simulink model "Simu_Autopilot_2015_updated"  (R2015a)
settings: Solver=ode15s  StartTime=0.0  StopTime=240  RelTol=1e-3
InitFcn:
  | clear all
  | addpath('../parameters/')
  | aircraft_parameters
  | simulation_parameters
  | wind_parameters
  | compute_autopilot_gains
undefined symbols (not defined in the file or in its folder): autopilot, drawAircraft, forces_moments, path_follow, path_manager, plotmavstatevariables, SIM, UAV, WIND
libraries: simulink x4
settings Model: CovHtmlReporting=off  CovSFcnEnable=off  Creator=beard  LastModifiedBy=User
settings DataIOCC: SignalLoggingSaveFormat=ModelDataLogs
settings OptimizationCC: ExpressionDepthLimit=2147483647  InitFltsAndDblsToZero=on
settings DebuggingCC: UnderspecifiedInitializationDetection=Classic  MergeDetectMultiDrivingBlocksExec=none  SolverPrmCheckMsg=warning  FcnCallInpInsideContextMsg=EnableAllAsWarning  StateNameClashWarn=warning
settings GRTTargetCC: CombineOutputUpdateFcns=off  GRTInterface=on

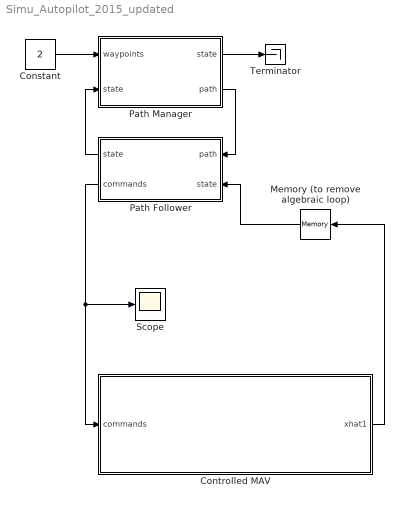
== system Simu_Autopilot_2015_updated ==
  Constant : Constant  Value=2
  Controlled MAV : Subsystem
  Memory (to remove algebraic loop) : Memory
  Path Follower : Subsystem
  Path Manager : Subsystem
  Scope : Scope
  Terminator : Terminator
  wires:
  Controlled MAV/1(xhat1) -> Memory (to remove algebraic loop)/1
  Memory (to remove algebraic loop)/1 -> Path Follower/2(state)
  Path Follower/2(commands) -> Scope/1, Controlled MAV/1(commands)
  Path Follower/1("state ") -> Path Manager/2(state)
  Path Manager/2(path) -> Path Follower/1(path)
  Constant/1 -> Path Manager/1(waypoints)
  Path Manager/1("state ") -> Terminator/1

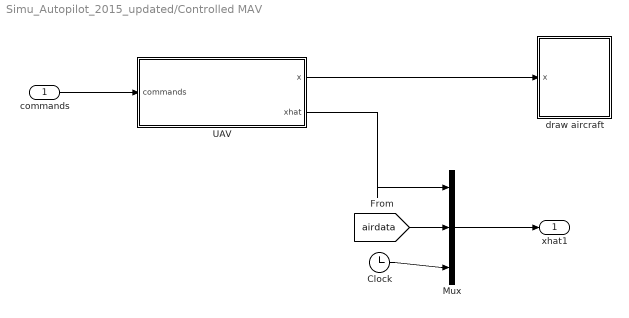
== system Simu_Autopilot_2015_updated/Controlled MAV ==
  commands : Inport
  Clock : Clock
  Mux : Mux  Inputs=3
  UAV : Subsystem
  draw aircraft : Subsystem
      mask Display: image(imread('tv.jpg'))
  xhat1 : Outport
  wires:
  commands/1 -> UAV/1(commands)
  UAV/1(x) -> draw aircraft/1(x)
  UAV/2(xhat) -> Mux/1
  [airdata] -> Mux/2
  Clock/1 -> Mux/3
  Mux/1 -> xhat1/1

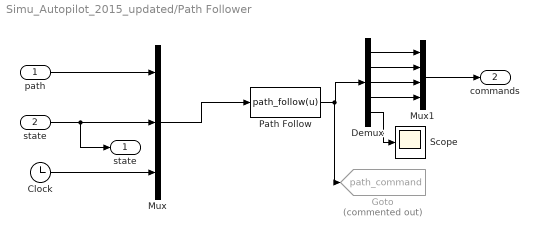
== system Simu_Autopilot_2015_updated/Path Follower ==
  path : Inport
  state : Inport  Port=2
  Clock : Clock
  Demux : Demux  Outputs=5
  Goto : Goto  Commented=on  GotoTag=path_command  TagVisibility=global
  Mux : Mux  Inputs=3
  Mux1 : Mux
  Path Follow : MATLABFcn  MATLABFcn=path_follow(u)  OutputDimensions=5
  Scope : Scope
  "state " : Outport
  commands : Outport  Port=2
  wires:
  Path Follow/1 -> Goto/1, Demux/1
  Demux/2 -> Mux1/2
  Demux/1 -> Mux1/1
  Demux/4 -> Mux1/4
  Clock/1 -> Mux/3
  Demux/5 -> Scope/1
  Demux/3 -> Mux1/3
  Mux1/1 -> commands/1
  path/1 -> Mux/1
  Mux/1 -> Path Follow/1
  state/1 -> "state "/1, Mux/2

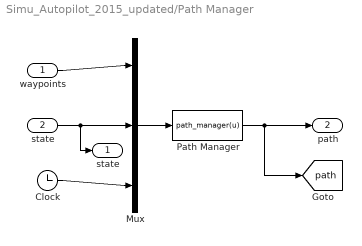
== system Simu_Autopilot_2015_updated/Path Manager ==
  waypoints : Inport
  state : Inport  Port=2
  Clock : Clock
  Mux : Mux  Inputs=3
  Path Manager : MATLABFcn  MATLABFcn=path_manager(u)  OutputDimensions=13
  "state " : Outport
  path : Outport  Port=2
  tag scope: path=global
  wires:
  Path Manager/1 -> path/1, [path]
  Mux/1 -> Path Manager/1
  waypoints/1 -> Mux/1
  Clock/1 -> Mux/3
  state/1 -> "state "/1, Mux/2

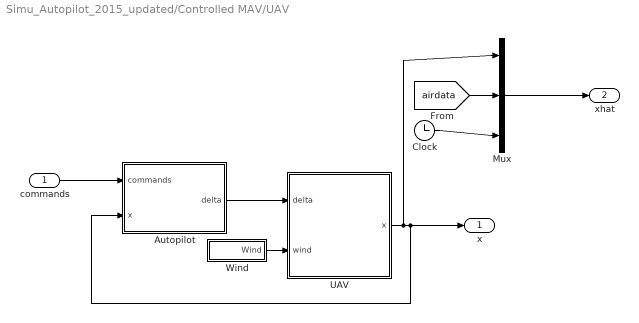
== system Simu_Autopilot_2015_updated/Controlled MAV/UAV ==
  commands : Inport
  Autopilot : Subsystem
      mask Display: image(imread('kestrel.jpg'))
  Clock : Clock
  Mux : Mux  Inputs=3
  UAV : Subsystem
      mask Display: image(imread('batcam.png'))
  Wind : Subsystem
  x : Outport
  xhat : Outport  Port=2
  wires:
  Wind/1(Wind) -> UAV/2(wind)
  Mux/1 -> xhat/1
  commands/1 -> Autopilot/1(commands)
  Autopilot/1(delta) -> UAV/1(delta)
  UAV/1(x) -> Mux/1, x/1, Autopilot/2(x)
  [airdata] -> Mux/2
  Clock/1 -> Mux/3

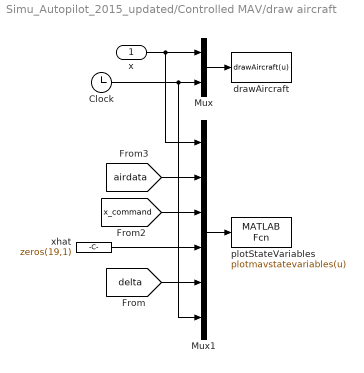
== system Simu_Autopilot_2015_updated/Controlled MAV/draw aircraft ==
  x : Inport
  Clock : Clock
  Mux : Mux  Inputs=2
  Mux1 : Mux  Inputs=6
  drawAircraft : MATLABFcn  MATLABFcn=drawAircraft(u)  OutputDimensions=0  SampleTime=SIM.ts_plotting
  plotStateVariables : MATLABFcn  MATLABFcn=plotmavstatevariables(u)  OutputDimensions=0  SampleTime=SIM.ts_plotting
  xhat : Constant  Value=zeros(19,1)
  wires:
  Mux/1 -> drawAircraft/1
  x/1 -> Mux1/1, Mux/1
  Clock/1 -> Mux1/6, Mux/2
  Mux1/1 -> plotStateVariables/1
  [x_command] -> Mux1/3
  [delta] -> Mux1/5
  [airdata] -> Mux1/2
  xhat/1 -> Mux1/4

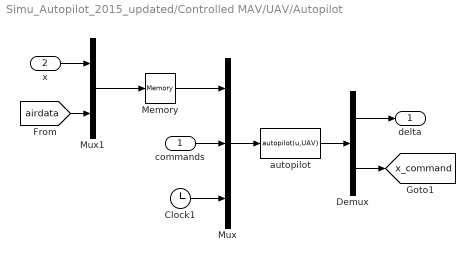
== system Simu_Autopilot_2015_updated/Controlled MAV/UAV/Autopilot ==
  commands : Inport
  x : Inport  Port=2
  Clock1 : Clock
  Demux : Demux  Outputs=[4;12]
  Memory : Memory
  Mux : Mux  Inputs=3
  Mux1 : Mux  Inputs=2
  autopilot : MATLABFcn  MATLABFcn=autopilot(u,UAV)  OutputDimensions=4+12  SampleTime=SIM.ts_simulation
  delta : Outport
  tag scope: x_command=global
  wires:
  Mux/1 -> autopilot/1
  autopilot/1 -> Demux/1
  Demux/1 -> delta/1
  Demux/2 -> [x_command]
  commands/1 -> Mux/2
  x/1 -> Mux1/1
  [airdata] -> Mux1/2
  Clock1/1 -> Mux/3
  Mux1/1 -> Memory/1
  Memory/1 -> Mux/1

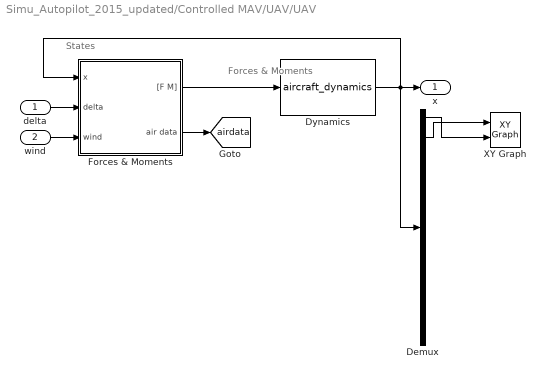
== system Simu_Autopilot_2015_updated/Controlled MAV/UAV/UAV ==
  note: Forces & Moments
  note: States
  delta : Inport
  wind : Inport  Port=2
  Demux : Demux  Outputs=12
  Dynamics : S-Function  FunctionName=aircraft_dynamics  Parameters=UAV
  Forces & Moments : Subsystem
  XY Graph : simulink/Sinks/XY Graph  xmin=-100  xmax=800  ymin=-400  ymax=400  st=-1
  x : Outport
  tag scope: airdata=global
  wires:
  Dynamics/1 -> Demux/1, Forces & Moments/1(x), x/1
  Forces & Moments/1("[F M]") -> Dynamics/1
  Forces & Moments/2(air data) -> [airdata]
  delta/1 -> Forces & Moments/2(delta)
  wind/1 -> Forces & Moments/3(wind)
  Demux/1 -> XY Graph/2
  Demux/2 -> XY Graph/1

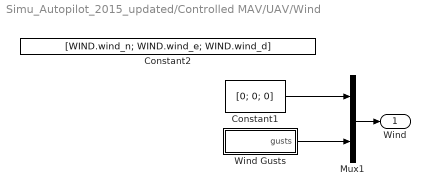
== system Simu_Autopilot_2015_updated/Controlled MAV/UAV/Wind ==
  Constant1 : Constant  Value=[0; 0; 0]
  Constant2 : Constant  Value=[WIND.wind_n; WIND.wind_e; WIND.wind_d]
  Mux1 : Mux  Inputs=2
  Wind Gusts : Subsystem
  Wind : Outport
  wires:
  Mux1/1 -> Wind/1
  Wind Gusts/1(gusts) -> Mux1/2
  Constant1/1 -> Mux1/1

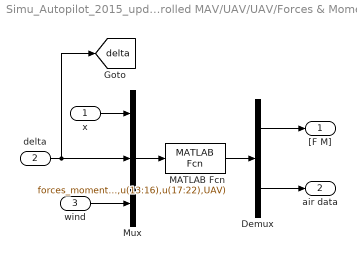
== system Simu_Autopilot_2015_updated/Controlled MAV/UAV/UAV/Forces & Moments ==
  x : Inport
  delta : Inport  Port=2
  wind : Inport  Port=3
  Demux : Demux  Outputs=[6;6]
  MATLAB Fcn : MATLABFcn  MATLABFcn=forces_moments(u(1:12),u(13:16),u(17:22),UAV)  OutputDimensions=12
  Mux : Mux  Inputs=3
  "[F M]" : Outport
  air data : Outport  Port=2
  tag scope: delta=global
  wires:
  Demux/2 -> air data/1
  Mux/1 -> MATLAB Fcn/1
  Demux/1 -> "[F M]"/1
  MATLAB Fcn/1 -> Demux/1
  wind/1 -> Mux/3
  delta/1 -> [delta], Mux/2
  x/1 -> Mux/1

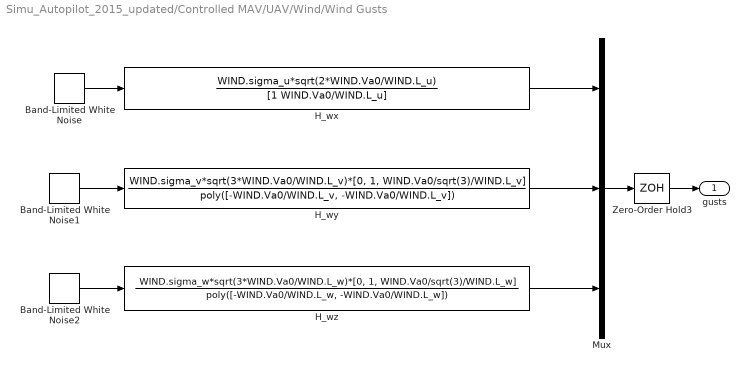
== system Simu_Autopilot_2015_updated/Controlled MAV/UAV/Wind/Wind Gusts ==
  Band-Limited White Noise : simulink/Sources/Band-Limited White Noise  Cov=[0.1]  Ts=SIM.ts_simulation  seed=[23341]
  Band-Limited White Noise1 : simulink/Sources/Band-Limited White Noise  Cov=[0.1]  Ts=SIM.ts_simulation  seed=[23341]
  Band-Limited White Noise2 : simulink/Sources/Band-Limited White Noise  Cov=[0.1]  Ts=SIM.ts_simulation  seed=[23341]
  H_wx : TransferFcn  Numerator=WIND.sigma_u*sqrt(2*WIND.Va0/WIND.L_u)  Denominator=[1 WIND.Va0/WIND.L_u]
  H_wy : TransferFcn  Numerator=WIND.sigma_v*sqrt(3*WIND.Va0/WIND.L_v)*[0, 1, WIND.Va0/sqrt(3)/WIND.L_v]  Denominator=poly([-WIND.Va0/WIND.L_v, -WIND.Va0/WIND.L_v])
  H_wz : TransferFcn  Numerator=WIND.sigma_w*sqrt(3*WIND.Va0/WIND.L_w)*[0, 1, WIND.Va0/sqrt(3)/WIND.L_w]  Denominator=poly([-WIND.Va0/WIND.L_w, -WIND.Va0/WIND.L_w])
  Mux : Mux  Inputs=3
  Zero-Order Hold3 : ZeroOrderHold  SampleTime=SIM.ts_simulation
  gusts : Outport
  wires:
  H_wx/1 -> Mux/1
  Band-Limited White Noise/1 -> H_wx/1
  H_wy/1 -> Mux/2
  Band-Limited White Noise1/1 -> H_wy/1
  H_wz/1 -> Mux/3
  Band-Limited White Noise2/1 -> H_wz/1
  Mux/1 -> Zero-Order Hold3/1
  Zero-Order Hold3/1 -> gusts/1
